simulink model "TrailerSoftware"  (R2019b)
settings: Solver=FixedStepDiscrete  StartTime=0.0  StopTime=inf  FixedStep=update  RelTol=1e-3  EnableMultiTasking=on
values from neighbouring files (symbols this model uses):
  countmax1 = 2500    [ProductionMfile.m]
  countmax2 = 2500    [ProductionMfile.m]
  HeaterIntGain = .0008    (= 0.0008)    [ProductionMfile.m]
  HeatGain = 10    [ProductionMfile.m]
  Intll = 0    [ProductionMfile.m]
  MaxCondPressure = 350    [ProductionMfile.m]
  MinSP = 1    [ProductionMfile.m]
  PostGain100 = 0.0002    [ProductionMfile.m]
  PostGain150 = 0.0005    [ProductionMfile.m]
  PostGain200 = 0.0004    [ProductionMfile.m]
  PostGain300 = 0.0008    [ProductionMfile.m]
  PostInit150 = 12    [ProductionMfile.m]
  PostIntulC = 65    [ProductionMfile.m]
  PostPGain = 0    [ProductionMfile.m]
  PreGain100 = 0.0005    [ProductionMfile.m]
  PreGain150 = 0.0005    [ProductionMfile.m]
  PreGain200 = 0.0003    [ProductionMfile.m]
  PreGain300 = 0.0008    [ProductionMfile.m]
  PreInit150 = 30    [ProductionMfile.m]
  PreIntulC = 65    [ProductionMfile.m]
  PreIntulDH = 65    [ProductionMfile.m]
  PrePGain = 0    [ProductionMfile.m]
  SatPress = [10 20 30 40 50 60 70 80 90 100 110 120 130 140 150 160 170      180 190 200 210 220 230 240 250 260 270 280 290 300 310 320 330      340 350 360 370 380 390 400 410 420 430 440 450 460 470 480 490      500]    [ProductionMfile.m]
  SatTemp = [-29.497 -2.4046 15.401 29.047 40.267 49.88 58.338 65.922 72.819      79.159 85.037 90.526 95.68 100.55 105.16 109.54 113.73 117.73 121.57      125.26 128.82 132.25 135.56 138.77 141.88 144.89 147.82 150.67 153.44      156.15 158.78 161.35 163.85 166.3 168.7 171.04 173.33 175.58 177.77      179.93 182.04 184.11 186.14 188.14 190.09 192.01 193.9 195.75 197.58      199.37]    [ProductionMfile.m]
  SHGain = 2    [ProductionMfile.m]
  SizeCANMatrix = 80    [ProductionMfile.m]
  SizeCOBIDVector = 10    [ProductionMfile.m]
  update = 0.002    [ProductionMfile.m]
undefined symbols (not defined in the file or in its folder): DiscIntNeverNeededParam, PostDGain, PreDGain, Ratio100, Ratio150, Ratio200, Ratio300
libraries: simulink x60, c2837xDlib x35, xpcutilitieslib x24, c2802xlib x8, c280xlib x7, etargetslib x4, svdutilitieslib x2, c2000lib x1
(part 8 of 8)

== matlab function TrailerSoftware/Subsystem/Display1 ==
  data: DisRow1 output; DisRow2 output; DisRow3 output; DisRow4 output; StartRow1 output; StartRow2 output; StartRow3 output; StartRow4 output; NumCharRow1 output; NumCharRow2 output; NumCharRow3 output; NumCharRow4 output; ClearDisplay output; DisplayDataAvail output; time input; MBV input; HeaterTempCom input; UseHeater input; CoolTempCom input; PressCommand input; warning1 input; warning2 input; warning3 input; fault1 input; fault2 input; fault3 input; Pulse input; FlowRate input; DuctTemp input; DuctPress input; DuctTempIn input; Hin input; Hout input
function [DisRow1,DisRow2,DisRow3,DisRow4,StartRow1,StartRow2,...
    StartRow3,StartRow4,NumCharRow1,NumCharRow2,NumCharRow3,NumCharRow4,...
    ClearDisplay,DisplayDataAvail]= fcn(time,MBV,...
    HeaterTempCom,UseHeater,CoolTempCom,PressCommand,warning1,warning2,warning3,fault1,fault2,...
    fault3,Pulse,FlowRate,DuctTemp,DuctPress,DuctTempIn,Hin,Hout)
persistent time0 count1 count2 displ  
if isempty(time0)
    time0 = time;
    count1 = 1;
    count2 = 1;
    displ = 0;
end
DisplayDataAvail = 0; %#ok<*NASGU>
if Pulse == 1
    DisplayDataAvail = 1;
end

TempCommand = CoolTempCom;
if UseHeater == 1
    TempCommand = HeaterTempCom;  
end
%#codegen
% MBV(1) = SystemStateValue;
%   Value  Name     Description 
%   0x0090 Menu     Controller is in the menu system
%   0x0093 Off      Controller is in the off mode
%   0x0096 Auto     Controller is in the auto mode
%   0x0099 Failure  Controller is in the failure mode
%   0x009C Running  Controller is in the running mode
% MBV(2) = RunningStateValue;
%   Value  Index        Name               Description
%   0x00   1            No Running         Mode Controller is not in any running state
%   0x01   2            Delay to Start     Controller is delaying to start
%   0x02   3            Preheat            Controller is preheating engine
%   0x03   4            Cranking           Controller is cranking engine
%   0x04   5            Crank Rest         Controller is resting before next crank
%   0x05   6            Crank Success      Controller has successfully started engine
%   0x06   7            Reserved           Reserved
%   0x07   8            Warmup             Controller is warming up engine before applying load
%   0x08   9            Running            Controller is in a normal running state
%   0x09   10           Cooldown           Controller is cooling down engine before shutting down
%   0x0A   11           Shutdown           Controller has shut down the engine
%   0x0B   12           Failure            Controller has shut down the engine due to a fault
%   0x20   13           Remote             Controller was started from 'Start / Stop' switched input
%   0x21   14           Manual             Controller was started from the front panel button
%   0x22   15           Modbus             Controller was started by Modbus command
%   0x23   16           Battery Recharge   Controller was started to recharge batteries
%   0x24   17           Exerciser          Controller was started from the exerciser clock
%   0x25   18           Auxiliary Sensor 1 Controller was started based on Auxiliary Sensor 1 reading
%   0x26   19           Auxiliary Sensor 2 Controller was started based on Auxiliary Sensor 2 reading
%   0x27   20           Loss of Mains      Controller was started due to loss of mains voltage
%   0x28   21           Momentary Switch   Controller was started from 'Momentary' switched input
%   0x29   22           Auxiliary Sensor 3 Controller was started based on Auxiliary Sensor 3 reading
%   0x2A   23           Auxiliary Sensor 4 Controller was started based on Auxiliary Sensor 4 reading
%    RunningState = MBV(2) + 1;


% MBV(3) = EventBitMap1ValueA;
%   Value  Description
%   0      Not In Auto Bit is on due to controller not being in auto mode
%   1      Idle Mode Bit is on due to controller being in idle mode
%   2      Battle Mode Bit is on due to controller being in battle mode
%   3      System OK Bit is on due to controller being free of warnings and failures
%   4      Glowplug Bit is on due to 'Preheat' timer
%   5      Warmup Bit is on due to 'Warmup' timer
%   6      Cooldown Bit is on due to 'Cooldown' timer
%   7      Engine Running Bit is on due to engine running
%   8      Exerciser Bit is on due to engine exercise
%   9      Battery Recharge Bit is on due to battery recharge
%   10     Maintenance Required Bit is on due to 'Maintenance Counter' timer expiring
%   11     Low Battery During Cranking Bit is on due to 'Low Battery Voltage During Cranking'
%   12     N/A
%   13     N/A
%   14     N/A
%   15     N/A 
    
% MBV(4) = EventBitMap1ValueB;
%   0      Delay to Start Bit is on due to 'Delay to Start' timer
%   1      Force Regeneration Bit is on due to a force regeneration (DPF)
%   2      Regeneration Inhibit Bit is on due to regeneration being inhibited (DPF)
%   3 ~ 7  Reserved Reserved
%   8      Fuel Bit is on due to fuel output enabled
%   9      Crank Bit is on due to crank output enabled
%   10     Genset Break1 Bit is on due to transferring to generator position
%   11     Mains Break1 Bit is on due to transferring to mains position
%   12     Pull Coil Bit is on due to pull coil being enabled
%   13     LCD Backlight Bit is on due to the LCD backlight being on
%   14     Voltage Regulator Bit is on when controller is not in idle mode
%   15     Energize to Stop Bit is on due to Energize to Stop timer
% MBV(5) = EventBitMap2ValueA;
%   0      Group Output 1 Bit is on due to output set to Group Output 1 is active
%   1      Group Output 2 Bit is on due to output set to Group Output 2 is active
%   2      Group Output 3 Bit is on due to output set to Group Output 3 is active
%   3      Group Output 4 Bit is on due to output set to Group Output 4 is active
%   4      Increment RPM Bit is on due to the RPM being manually incremented through speed
%          control
%   5      Decrement RPM Bit is on due to the RPM being manually decremented through speed
%          control
%   6      DEF Fluid Pump Bit is on due to DEF Fluid Pump being on
%   7      Genset Disable Bit is on due to the Genset being disabled
%   8      Dummy Load ON Bit is on due to Dummy Load being enabled
%   9 ~ 11 Reserved Reserved
%   12     Glowplug Bit is on due to preheat input or ECM preheat being active
%   13     Common Fault Bit is on due to a any fault occurring
%   14     Temperature Unit Reserved - Fixed to Fahrenheit
%   15     Pressure Unit Reserved - Fixed to PSI
% MBV(6) = EventBitMap2ValueB;
%   0      Overcrank Warning Bit is on due to controller failing to crank engine on first attempt
%   1      Invalid Setting Warning Bit is on due to an invalid setting being stored in the controller
%   2      Emergency Input Bit is on due to Emergency Stop input being active
%   3      EPS Load is On Bit is on due to current readings being at least 5% of the rated current
%          setting
%   4      Genset Break On1 Reserved
%   5      Mains Break On1 Reserved
%   6      Mains Pickup1 Bit is on due to mains voltage being within acceptable levels after
%          dropping out
%   7      Mains Dropout1 Bit is on due to controller sensing mains voltage has dropped out
%   8      Mains OK1 Bit is on due to mains voltage being within acceptable levels
%   9      Start Inhibit Bit is on due to Start Inhibit input being active
%   10     Remote Reset Bit is on due to the Remote Reset input being active
%   11 ~15 N/A
% MBV(7) = FaultBitMapValueA;
%   Bit   Name                  Description
%   0     Overcrank             Fault due to max attempts at cranking
%   without starting (1)
%   1     Engine Failed to Stop Fault due to engine speed not being 0 RPM
%   at shutdown (2)
%   2     DM1 Stop Lamp1        DM1 Stop Lamp is on (not used) (3)
%   3     High Engine Temp      Fault due to high engine temperature (4)
%   4     Low Oil Pressure      Fault due to low oil pressure (5)
%   5     Low Fuel Level        Fault due to low fuel level (6)
%   6     Under Speed           Fault due to low engine speed (7)
%   7     Over Speed            Fault due to high engine speed (8)
%   8     Low Battery Voltage   Fault due to low battery voltage (9)
%   9     High Battery Voltage  Fault due to high battery voltage (10)
%   10    Low Coolant Level     Fault due to low coolant level (11)
%   11    Low Air Pressure      Fault due to low air pressure (not used)
%   (12)
%   12    Low Hydraulic Press   Fault due to low hydraulic pressure (not
%   used) (13)
%   13    Under Frequency       Fault due to low AC frequency (14)
%   14    Over Frequency        Fault due to high AC frequency (15)
%   15    AC Under Voltage      Fault due to low AC voltage (16)
% MBV(8) = FaultBitMapValueB;
%   0     AC Over Voltage       Fault due to high AC voltage (17)
%   1     ECM Communication     Fault due to loss of communications with
%   ECM (18)
%   2     Configurable Failure 1 Fault due to Configurable Fail Input 1
%   being active (not used) (19)
%   3     Configurable Failure 2 Fault due to Configurable Fail Input 2
%   being active (not used) (20)
%   4     Auxiliary Sensor 1    Fault due to low / high reading on
%   Auxiliary Sensor 1  (not used) (21)
%   5     Auxiliary Sensor 2    Fault due to low / high reading on
%   Auxiliary Sensor 2 (not used) (22)
%   6     Auxiliary Sensor 3    Fault due to low / high reading on Auxiliary Sensor 3 
%   (not used) (23)
%   7     Auxiliary Sensor 4    Fault due to low / high reading on
%   Auxiliary Sensor 4 (not used) (24)
%   8     Over Current          Fault due to high current reading (25)
%   9     Configurable Failure 3 Fault due to Configurable Fail Input 3
%   being active (not used) (26)
%   26 ~ 31 Reserved Reserved (not used) (27-32)
       
%   Bit   Name                  Description
%   0     Low Engine Temp       Warning due to low engine temperature
%   1     High Engine Temp      Warning due to high engine temperature
%   2     Low Oil Pressure      Warning due to low oil pressure
%   3     Under Speed           Warning due to low engine speed
%   4     Over Speed            Warning due to high engine speed
%   5     Low Fuel Level        Warning due to low fuel level
%   6     High Fuel Level       Warning due to high fuel level
%   7     Low Battery Voltage   Warning due to low battery voltage
%   8     High Battery Voltage  Warning due to high battery voltage
%   9     Under Frequency       Warning due to low AC frequency
%   10    Over Frequency        Warning due to high AC frequency
%   11    AC Under Voltage      Warning due to low AC voltage
%   12    AC Over Voltage       Warning due to high AC voltage
%   13    Battery Charger Fault Warning due to battery charger fault
%   14    Over Current          Warning due to high AC current
%   15    Fuel In Basin         Warning due to fuel being in the catch basin
% MBV(10) = WarningBitMapValueB;
%   Bit   Name                  Description
%   0     Configurable Warning 1 Warning due to Configurable Warn Input 1 being active
%   1     Configurable Warning 2 Warning due to Configurable Warn Input 2 being active
%   2     Auxiliary Sensor 1     Warning due to low / high reading on Auxiliary Sensor 1
%   3     Auxiliary Sensor 2     Warning due to low / high reading on Auxiliary Sensor 2
%   4     Auxiliary Sensor 3     Warning due to low / high reading on Auxiliary Sensor 3
%   5     Auxiliary Sensor 4     Warning due to low / high reading on Auxiliary Sensor 4
%   6 ~ 15 Reserved Reserved
% MBV(11) = GenFreqValue;
% MBV(12) = GenVoltValueA;
% MBV(13) = GenVoltValueB;
% MBV(14) = GenVoltValueC;
% MBV(15) = GenCurValueA;
% MBV(16) = GenCurValueB;
% MBV(17) = GenCurValueC;
% MBV(18) = EngineTempValue;
% MBV(19) = EngineOilPressValue;
% MBV(20) = FuelLevelValue;
% MBV(21) = BatteryVoltValue;
% MBV(22) = EngineRunHoursValue;
% MBV(23) = FCSuperHeatValue;
% MBV(24) = RCSuperHeatValue;
% MBV(25) = SuctionPressValue;
% MBV(26) = FSatTempValue;
% MBV(27) = RSatTempValue;
% MBV(28) = FSucTempValue;
% MBV(29) = RSucTempValue;
% MBV(30) = FRmTempValue;
% MBV(31) = RRmTempValue;
% MBV(32) = FValPosValue;
% MBV(33) = RValPosValue;
% MBV(34) = FEvapTempValue;
% MBV(35) = REvapTempValue;
% MBV(36) = FAlarmValue;
% MBV(37) = RAlarmValue;

FuelLevelValue = MBV(20);
s1 = convertnum(FuelLevelValue);
s2 = convertnum(FlowRate);
s6 = convertnum(min(140,max(TempCommand,0)));
s7 = convertnum(min(9,max(PressCommand,0)));
s8 = convertnum(min(140,max(DuctTemp,0)));
s9 = convertnum(min(9,max(DuctPress,0)));
s10 = convertnum(min(140,max(DuctTempIn,0)));
s11 = convertnum(min(99,max(Hin,0)));
s12 = convertnum(min(99,max(Hout,0)));
Message1 = ['TempSet ' s6(1:3)...
    ',Meas' s8(1:3) 'F'];
Message2 = ['PSet' s7(1:4)...
    ',Meas' s9(1:4) 'psi'];
Message3 = ['Inlet Air Temp: ' s10...
    ', deg F  ','Fuel Level ' s1...
    ',% ' 'Humidity Inlet ' s11...
    ',% ' 'Humidity Outlet ' s12...
    ',% '  'Flow Rate Selected = ' s2...
    ', lbm/min'];
    
s4A = convertnum(min(999,max(warning1,0)));
s4B = convertnum(min(999,max(warning2,0)));
s4C = convertnum(min(999,max(warning3,0)));
s5A = convertnum(min(999,max(fault1,0)));
s5B = convertnum(min(999,max(fault2,0)));
s5C = convertnum(min(999,max(fault3,0)));

 Message4 = [' Warning = ' s4A ' ' s4B ' ' s4C ' Fault = ' s5A...
        ' ' s5B ' ' s5C ' '];

DisRow1 = uint8(32*ones(20,1));
DisRow2 = uint8(32*ones(20,1));
DisRow3 = uint8(32*ones(20,1));
DisRow4 = uint8(32*ones(20,1));
StartRow1 = uint8(1);
StartRow2 = uint8(1);
StartRow3 = uint8(1);
StartRow4 = uint8(1);
NumCharRow1 = uint8(20);
NumCharRow2 = uint8(20);
NumCharRow3 = uint8(20);
NumCharRow4 = uint8(20);
ClearDisplay = uint8(0);
DisplayDataAvail = uint8(0);
if displ == 1
    DisplayDataAvail = uint8(1);
    displ = 0;
end
if time > time0 + .5
    time0 = time;
    displ = 1;
    count1 = count1 + 1;
    count2 = count2 + 1;
    if count1 == length(Message3) - 20
        count1 = 1;
    end
    if count2 == length(Message4) - 20
        count2 = 1;
    end
end
    
DisRow1(:,1) = Message1;
DisRow2(:,1) = Message2;
DisRow3(:,1) = Message3(1,count1:count1+19)';
DisRow4(:,1) = Message4(1,count2:count2+19)';

return

% Convert number to string
function y = convertnum(input)
    y = uint8(32*ones(1,5));
    int_part = double(floor(input));
    float_part = input - double(int_part);
    i = 1;
    temp = int_part;
    if temp < 10
        y(i) = uint8(temp + 48);  
        i = 2;
    elseif floor(temp/10) < 10
        y(i) = uint8(floor(temp/10)+48);
        y(i+1) = uint8((temp - floor(temp/10)*10) + 48);
        i = 3;
    elseif floor(temp/100) < 10
        y(i) = uint8(floor(temp/100)+48);
        y(i+1) = uint8(floor((temp - floor(temp/100)*100)/10) + 48);
        y(i+2) = uint8((temp - floor(temp/10)*10) + 48);
        i = 4;
    end
    y(i) = '.';
    temp = float_part;
    i = i + 1;
    if temp*10 < 10
        y(i) = uint8((temp*10) + 48);  
    end
    
return
